simulink model "suspension"  (R2020a)
settings: Solver=VariableStepAuto  StartTime=0.0  StopTime=40  RelTol=1e-3
undefined symbols (not defined in the file): alfa, beta, cc, cw, dc, dw, k, mc, mw
settings Model: Creator=bnier  LastModifiedBy=bnier

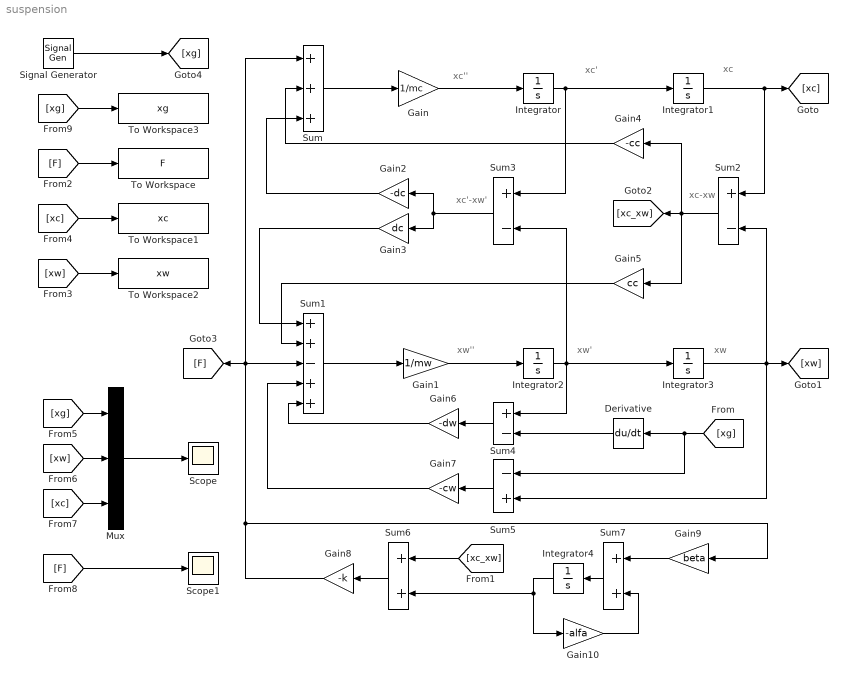
== system suspension ==
  note: xc'-xw'
  note: xc-xw
  note: xw
  note: xw'
  note: xw''
  note: xc
  note: xc'
  note: xc''
  Derivative : Derivative
  Gain : Gain  Gain=1/mc
  Gain1 : Gain  Gain=1/mw
  Gain10 : Gain  Gain=-alfa
  Gain2 : Gain  Gain=-dc
  Gain3 : Gain  Gain=dc
  Gain4 : Gain  Gain=-cc
  Gain5 : Gain  Gain=cc
  Gain6 : Gain  Gain=-dw
  Gain7 : Gain  Gain=-cw
  Gain8 : Gain  Gain=-k
  Gain9 : Gain  Gain=beta
  Integrator{,1..4} (5 alike) : Integrator
  Mux : Mux  Inputs=3
  Scope : Scope
  Scope1 : Scope
  Signal Generator : SignalGenerator  WaveForm=square  Amplitude=0.2  Frequency=0.05
  Sum : Sum  Inputs=+++
  Sum1 : Sum  Inputs=++-++
  Sum2 : Sum  Inputs=+-
  Sum3 : Sum  Inputs=+-
  Sum4 : Sum  Inputs=+-
  Sum5 : Sum  Inputs=-+
  Sum6 : Sum
  Sum7 : Sum
  To Workspace : ToWorkspace  VariableName=F  SaveFormat=Timeseries  SampleTime=-1
  To Workspace1 : ToWorkspace  VariableName=xc  SaveFormat=Timeseries  SampleTime=-1
  To Workspace2 : ToWorkspace  VariableName=xw  SaveFormat=Timeseries  SampleTime=-1
  To Workspace3 : ToWorkspace  VariableName=xg  SaveFormat=Timeseries  SampleTime=-1
  wires:
  Sum/1 -> Gain/1
  Gain/1 -> Integrator/1
  Integrator/1 -> Sum3/1, Integrator1/1
  Integrator1/1 -> [xc], Sum2/1
  Integrator2/1 -> Sum4/1, Integrator3/1, Sum3/2
  Integrator3/1 -> [xw], Sum5/2, Sum2/2
  Sum1/1 -> Gain1/1
  Gain1/1 -> Integrator2/1
  Sum2/1 -> Gain4/1, [xc_xw], Gain5/1
  Sum3/1 -> Gain3/1, Gain2/1
  Gain2/1 -> Sum/3
  Gain3/1 -> Sum1/1
  Gain4/1 -> Sum/2
  Gain5/1 -> Sum1/2
  Sum4/1 -> Gain6/1
  Gain6/1 -> Sum1/5
  Derivative/1 -> Sum4/2
  [xg] -> Sum5/1, Derivative/1
  Sum5/1 -> Gain7/1
  Gain7/1 -> Sum1/4
  Sum6/1 -> Gain8/1
  [xc_xw] -> Sum6/1
  Gain8/1 -> Gain9/1, [F], Sum/1, Sum1/3
  Gain9/1 -> Sum7/1
  Sum7/1 -> Integrator4/1
  Integrator4/1 -> Sum6/2, Gain10/1
  Gain10/1 -> Sum7/2
  [xw] -> To Workspace2/1
  [xc] -> To Workspace1/1
  [F] -> To Workspace/1
  Mux/1 -> Scope/1
  [xg] -> Mux/1
  [xc] -> Mux/3
  [xw] -> Mux/2
  Signal Generator/1 -> [xg]
  [F] -> Scope1/1
  [xg] -> To Workspace3/1
